simulink model "PID_revised6"  (R2015a)
settings: Solver=ode45  StartTime=0.0  StopTime=1  RelTol=1e-3
libraries: simulink x1, powerlib_meascontrol x1
settings Model: Creator=Prasenjit Chandra  LastModifiedBy=Pranabendra

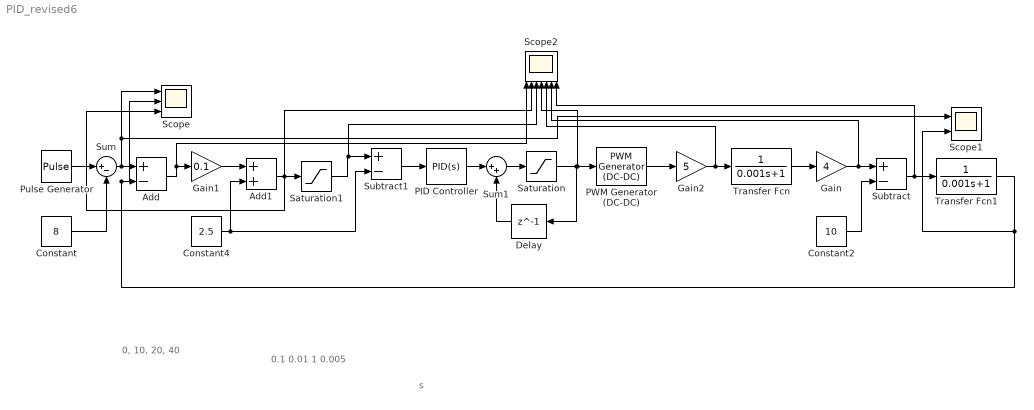
== system PID_revised6 ==
  note: 0.1 0.01
      | 1 0.005
  note: s
  note: 0, 10, 20, 40
  Add : Sum  Inputs=+-
  Add1 : Sum
  Constant : Constant  Value=8
  Constant2 : Constant  Value=10
  Constant4 : Constant  Value=2.5
  Delay : Delay  DelayLength=1  InitialCondition=0  SampleTime=0.0002
  Gain : Gain  Gain=4
  Gain1 : Gain  Gain=0.1
  Gain2 : Gain  Gain=5
  PID Controller : simulink/Continuous/PID Controller  Controller=PID  TimeDomain=Continuous-time  SampleTime=-1  IntegratorMethod=Forward Euler  FilterMethod=Forward Euler  Form=Parallel  UseFilter=on  ControllerParametersSource=internal  P=0.02  I=0.005  D=0  N=100  InitialConditionSource=internal  InitialConditionForIntegrator=0  InitialConditionForFilter=0  ExternalReset=none  LimitOutput=off  UpperSaturationLimit=inf  LowerSaturationLimit=-inf  LinearizeAsGain=on  AntiWindupMode=none  Kb=1  TrackingMode=off  Kt=1  PParamMin=[]  PParamMax=[]  IParamMin=[]  IParamMax=[]  DParamMin=[]  DParamMax=[]  NParamMin=[]  NParamMax=[]  KbParamMin=[]  KbParamMax=[]  KtParamMin=[]  KtParamMax=[]  POutMin=[]  POutMax=[]  IOutMin=[]  IOutMax=[]  DOutMin=[]  DOutMax=[]  NOutMin=[]  NOutMax=[]  KbOutMin=[]  KbOutMax=[]  KtOutMin=[]  KtOutMax=[]  IntegratorOutMin=[]  IntegratorOutMax=[]  FilterOutMin=[]  FilterOutMax=[]  SumOutMin=[]  SumOutMax=[]  SumI1OutMin=[]  SumI1OutMax=[]  SumI2OutMin=[]  SumI2OutMax=[]  SumI3OutMin=[]  SumI3OutMax=[]  SumDOutMin=[]  SumDOutMax=[]  SaturationOutMin=[]  SaturationOutMax=[]  IntegratorContinuousStateAttributes=''  IntegratorStateMustResolveToSignalObject=off  IntegratorRTWStateStorageClass=Auto  FilterContinuousStateAttributes=''  FilterStateMustResolveToSignalObject=off  FilterRTWStateStorageClass=Auto  DifferentiatorICPrevScaledInput=0  DifferentiatorOutMin=[]  DifferentiatorOutMax=[]
  PWM Generator (DC-DC) : powerlib_meascontrol/Pulse & Signal Generators/PWM Generator (DC-DC)  Fsw=5000  Ts=0
  Pulse Generator : DiscretePulseGenerator  PulseType=Time based  Amplitude=16  Period=1/10  PulseWidth=50
  Saturation : Saturate  UpperLimit=0.995  LowerLimit=0.005
  Saturation1 : Saturate  UpperLimit=4.95  LowerLimit=0.05
  Scope : Scope  NumInputPorts=3
      settings: YMin=-5~-5~-5  YMax=5~5~5
  Scope1 : Scope  NumInputPorts=2
      settings: YMin=-5~-5  YMax=5~5
  Scope2 : Scope  NumInputPorts=7
      settings: YMin=-5~-5~-5~-5~-5~-5~-5  YMax=5~5~5~5~5~5~5  SaveName=ScopeData2
  Subtract : Sum  Inputs=+-
  Subtract1 : Sum  Inputs=+-
  Sum : Sum  Inputs=|+-
  Sum1 : Sum  Inputs=|++
  Transfer Fcn : TransferFcn  Denominator=[0.001 1]
  Transfer Fcn1 : TransferFcn  Denominator=[0.001 1]
  wires:
  Pulse Generator/1 -> Sum/1
  Constant/1 -> Sum/2
  Saturation/1 -> Delay/1, PWM Generator (DC-DC)/1, Scope2/4
  Gain/1 -> Scope2/6, Subtract/1
  Sum/1 -> Scope1/1, Scope/1, Add/1
  Transfer Fcn/1 -> Gain/1
  Constant2/1 -> Subtract/2
  Sum1/1 -> Saturation/1
  PID Controller/1 -> Sum1/1
  Delay/1 -> Sum1/2
  Add/1 -> Scope2/1, Gain1/1
  Gain1/1 -> Add1/1
  Subtract1/1 -> PID Controller/1
  Saturation1/1 -> Scope2/3, Subtract1/1
  Constant4/1 -> Subtract1/2, Add1/2
  Subtract/1 -> Transfer Fcn1/1, Scope2/7
  PWM Generator (DC-DC)/1 -> Gain2/1
  Gain2/1 -> Scope2/5, Transfer Fcn/1
  Add1/1 -> Scope2/2, Scope/3, Saturation1/1
  Transfer Fcn1/1 -> Scope1/2, Scope/2, Add/2
